simulink model "scattering_pos_pos_old"  (R2022b)
settings: Solver=VariableStepAuto  StartTime=0.0  StopTime=10.0  RelTol=1e-3
values from neighbouring files (symbols this model uses):
  A = 2    [scattering_params.m]    (also in scattering_params_force_pos.m = 3; scattering_params_pos_pos.m = 3)
  b = 1    [scattering_params.m]    (also in scattering_params_force_pos.m = 40; scattering_params_pos_pos.m = 100)
  Be = 100    [scattering_params.m]    (also in scattering_params_force_pos.m; scattering_params_pos_pos.m)
  Bh = 1.5    [scattering_params.m]    (also in scattering_params_force_pos.m = 1; scattering_params_pos_pos.m = 1)
  Dh = 0.1    [scattering_params.m]    (also in scattering_params_force_pos.m = 16; scattering_params_pos_pos.m = 16)
  discrete_delay = 100    [scattering_params_force_pos.m]    (also in scattering_params_pos_pos.m)
  Fc = 1    [scattering_params.m]    (also in scattering_params_force_pos.m = 0.25; scattering_params_pos_pos.m = 0.25)
  Flp = 5    [scattering_params.m]    (also in scattering_params_force_pos.m = 0.5; scattering_params_pos_pos.m = 0.5)
  Jh = 1    [scattering_params.m]    (also in scattering_params_force_pos.m; scattering_params_pos_pos.m)
  Ke = 200    [scattering_params.m]    (also in scattering_params_force_pos.m; scattering_params_pos_pos.m)
  Mm = 0.5    [scattering_params.m]    (also in scattering_params_force_pos.m; scattering_params_pos_pos.m)
  Ms = 2    [scattering_params.m]    (also in scattering_params_force_pos.m; scattering_params_pos_pos.m)
  Ph = 10    [scattering_params.m]    (also in scattering_params_force_pos.m; scattering_params_pos_pos.m)
  scattering_filter_freq = 10    [scattering_params.m]    (also in scattering_params_force_pos.m; scattering_params_pos_pos.m)
  Ts = 0.001    [scattering_params_force_pos.m]    (also in scattering_params_pos_pos.m)
  xe = 5    [scattering_params.m]    (also in scattering_params_force_pos.m = 2; scattering_params_pos_pos.m = 2)
settings Model: Creator=Manu  LastModifiedBy=Manu

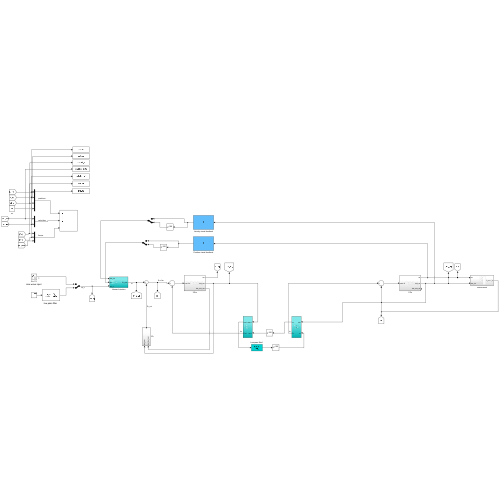
[thumbnail: Simulink's stored preview of the top-level diagram]
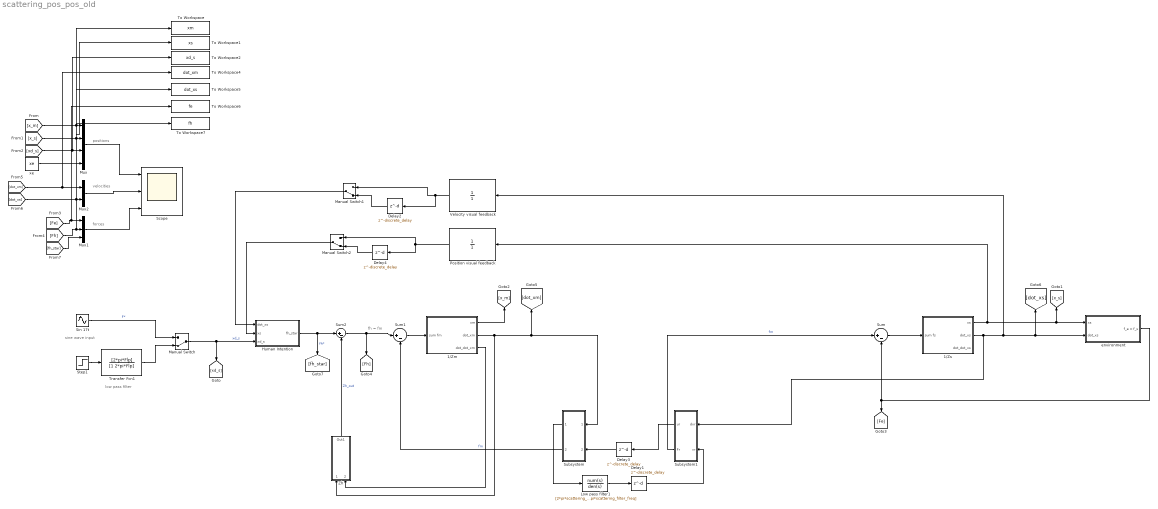
== system scattering_pos_pos_old ==
  note: fh = fm
  note: sine wave input
  note: low pass filter
  note: positions
  note: forces
  note: velocities
  1/Zm : Subsystem
  1/Zs : Subsystem
  Delay{1..4} (4 alike) : Delay  DelayLength=discrete_delay  SampleTime=Ts
  Human Intention : Subsystem
  Low pass filter1 : TransferFcn  Numerator=[2*pi*scattering_filter_freq]  Denominator=[1 2*pi*scattering_filter_freq]
  Manual Switch : ManualSwitch  CurrentSetting=0
  Manual Switch1 : ManualSwitch  CurrentSetting=0
  Manual Switch2 : ManualSwitch  CurrentSetting=0
  Mux : Mux
  Mux1 : Mux  Inputs=3
  Mux2 : Mux  Inputs=2
  Position visual feedback : TransferFcn  Denominator=[1]
  Scope : Scope  NumInputPorts=3
  Sin 17t : Sin  Amplitude=A  Frequency=2*pi*Fc  SampleTime=0
  Step1 : Step  Time=0.5  After=A  SampleTime=0
  Subsystem : Subsystem
      settings: PortSchema="{\"entries\":[{\"content\":{\"sides\":[{\"content\":{\"connectorIds\":[\"Out1\",\"Out2\"]},\"type\":\"ConnectorPlacement.EquallySpacedRectSide\",\"uuid\":\"82be490b-f4e1-4469-8bd6-488a0e070f91\"},{\"content\":{\"connectorIds\":[\"In1\",\"In2\"],\"side\":\"RIGHT\"},\"type\":\"ConnectorPlacement.EquallySpacedRectSide\",\"uuid\":\"c4a13bf6-21c5-475e-be70-cb3636e820b8\"},{\"content\":{\"connectorIds\":[],\"side\":\"TOP\"},\"type\":\"ConnectorPlacement.EquallySpacedRectSide\",\"uuid\":\"239945ea-98d9-43ca-9337-d0acd489fa2c\"},{\"content\":{\"connectorIds\":[],\"side\":\"HIDDEN\"},\"type\":\"ConnectorPlacement.EquallySpacedRectSide\",\"uuid\":\"ab55d6c9-2d6b-496a-b62d-f74546630c92\"}]},\"type\":\"ConnectorPlacement.EquallySpacedConnector\",\"uuid\":\"f2ee4140-76ed-4153-9f7f-3580e67d072a\"}],\"packageUris\":[\"http://schema.mathworks.com/mf0/Connector/R2020b\"],\"version\":\"1.0\"}"
  Subsystem1 : Subsystem
      settings: PortSchema="{\"entries\":[{\"content\":{\"sides\":[{\"content\":{\"connectorIds\":[\"Out1\",\"Out2\"]},\"type\":\"ConnectorPlacement.EquallySpacedRectSide\",\"uuid\":\"82be490b-f4e1-4469-8bd6-488a0e070f91\"},{\"content\":{\"connectorIds\":[\"In1\",\"In2\"],\"side\":\"RIGHT\"},\"type\":\"ConnectorPlacement.EquallySpacedRectSide\",\"uuid\":\"c4a13bf6-21c5-475e-be70-cb3636e820b8\"},{\"content\":{\"connectorIds\":[],\"side\":\"TOP\"},\"type\":\"ConnectorPlacement.EquallySpacedRectSide\",\"uuid\":\"239945ea-98d9-43ca-9337-d0acd489fa2c\"},{\"content\":{\"connectorIds\":[],\"side\":\"HIDDEN\"},\"type\":\"ConnectorPlacement.EquallySpacedRectSide\",\"uuid\":\"ab55d6c9-2d6b-496a-b62d-f74546630c92\"}]},\"type\":\"ConnectorPlacement.EquallySpacedConnector\",\"uuid\":\"f2ee4140-76ed-4153-9f7f-3580e67d072a\"}],\"packageUris\":[\"http://schema.mathworks.com/mf0/Connector/R2020b\"],\"version\":\"1.0\"}"
  Sum : Sum  Inputs=|+-
  Sum1 : Sum  Inputs=|+-
  Sum2 : Sum  Inputs=|+-
  To Workspace : ToWorkspace  VariableName=xm  SaveFormat=Timeseries  SampleTime=-1
  To Workspace1 : ToWorkspace  VariableName=xs  SaveFormat=Timeseries  SampleTime=-1
  To Workspace2 : ToWorkspace  VariableName=xd_s  SaveFormat=Timeseries  SampleTime=-1
  To Workspace4 : ToWorkspace  VariableName=dot_xm  SaveFormat=Timeseries  SampleTime=-1
  To Workspace5 : ToWorkspace  VariableName=dot_xs  SaveFormat=Timeseries  SampleTime=-1
  To Workspace6 : ToWorkspace  VariableName=fe  SaveFormat=Timeseries  SampleTime=-1
  To Workspace7 : ToWorkspace  VariableName=fh  SaveFormat=Timeseries  SampleTime=-1
  Transfer Fcn1 : TransferFcn  Numerator=[2*pi*Flp]  Denominator=[1 2*pi*Flp]
  Velocity visual feedback : TransferFcn  Denominator=[1]
  Zh : Subsystem
  environment : Subsystem
  xe : Constant  Value=xe
  wires:
  1/Zm/1(xm) -> [x_m]
  Manual Switch/1 -> [xd_s], Human Intention/3(xd_s)  "xd_s"
  Zh/1(Out1) -> Sum2/2  "Zh_out"
  Sin 17t/1 -> Manual Switch/1  "F*"
  1/Zm/3(dot_dot_xm) -> Zh/2(dot_dot_xm)
  Human Intention/1(fh_star) -> Sum2/1, [fh_star]  "fh*"
  Transfer Fcn1/1 -> Manual Switch/2
  Step1/1 -> Transfer Fcn1/1
  Sum2/1 -> [Fh], Sum1/1
  Sum1/1 -> 1/Zm/1(sum fm)
  Sum/1 -> 1/Zs/1(sum fs)
  1/Zs/2(dot_xs) -> Subsystem1/1(dxr), Velocity visual feedback/1, [dot_xs], environment/2(dot_xs)
  1/Zs/1(xs) -> [x_s], environment/1(xs), Position visual feedback/1
  environment/1(f_e = f_s) -> [Fe], Sum/2
  Velocity visual feedback/1 -> Delay2/1, Manual Switch1/1
  Manual Switch1/1 -> Human Intention/1(dot_xs)
  Delay4/1 -> Manual Switch2/2
  Position visual feedback/1 -> Delay4/1, Manual Switch2/1
  Manual Switch2/1 -> Human Intention/2(xs)
  1/Zm/2(dot_xm) -> Subsystem/1(dxm1), [dot_xm], Zh/1(dot_xm)
  Subsystem/2(Fm1) -> Sum1/2  "fm"
  Subsystem1/2(Fr) -> Sum/1  "fm"
  Subsystem/1(um1) -> Low pass filter1/1
  Subsystem1/1(ur) -> Delay3/1
  Low pass filter1/1 -> Delay1/1
  Delay2/1 -> Manual Switch1/2
  Delay3/1 -> Subsystem/2(vm1)
  Delay1/1 -> Subsystem1/2(vr)
  [fh_star] -> Mux1/3
  Mux2/1 -> Scope/2
  [Fh] -> To Workspace7/1, Mux1/2
  [dot_xs] -> To Workspace5/1, Mux2/2
  [dot_xm] -> Mux2/1, To Workspace4/1
  [x_s] -> To Workspace1/1, Mux/2
  [x_m] -> To Workspace/1, Mux/1
  Mux1/1 -> Scope/3
  Mux/1 -> Scope/1
  xe/1 -> Mux/4
  [Fe] -> Mux1/1, To Workspace6/1
  [xd_s] -> To Workspace2/1, Mux/3

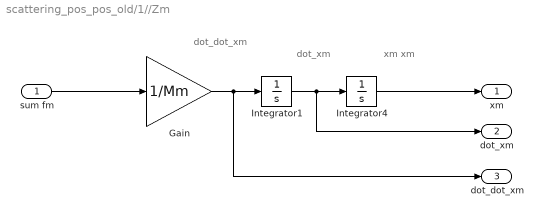
== system scattering_pos_pos_old/1//Zm ==
  note: dot_dot_xm
  note: dot_xm
  note: xm
      | xm
  sum fm : Inport
  Gain : Gain  Gain=1/Mm
  Integrator1 : Integrator
  Integrator4 : Integrator
  xm : Outport
  dot_xm : Outport  Port=2
  dot_dot_xm : Outport  Port=3
  wires:
  sum fm/1 -> Gain/1
  Gain/1 -> dot_dot_xm/1, Integrator1/1
  Integrator4/1 -> xm/1
  Integrator1/1 -> dot_xm/1, Integrator4/1

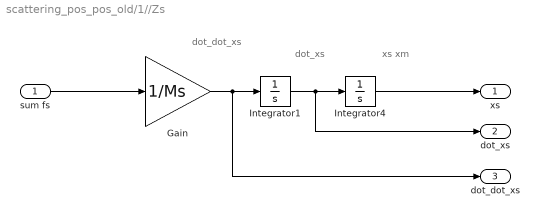
== system scattering_pos_pos_old/1//Zs ==
  note: dot_dot_xs
  note: dot_xs
  note: xs
      | xm
  sum fs : Inport
  Gain : Gain  Gain=1/Ms
  Integrator1 : Integrator
  Integrator4 : Integrator
  xs : Outport
  dot_xs : Outport  Port=2
  dot_dot_xs : Outport  Port=3
  wires:
  sum fs/1 -> Gain/1
  Gain/1 -> dot_dot_xs/1, Integrator1/1
  Integrator4/1 -> xs/1
  Integrator1/1 -> dot_xs/1, Integrator4/1

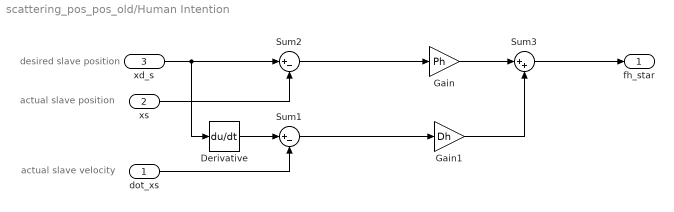
== system scattering_pos_pos_old/Human Intention ==
  note: actual slave velocity
  note: actual slave position
  note: desired slave position
  dot_xs : Inport
  xs : Inport  Port=2
  xd_s : Inport  Port=3
  Derivative : Derivative
  Gain : Gain  Gain=Ph
  Gain1 : Gain  Gain=Dh
  Sum1 : Sum  Inputs=|+-
  Sum2 : Sum  Inputs=|+-
  Sum3 : Sum  Inputs=|++
  fh_star : Outport
  wires:
  xs/1 -> Sum2/2
  dot_xs/1 -> Sum1/2
  Sum2/1 -> Gain/1
  Sum1/1 -> Gain1/1
  Gain1/1 -> Sum3/2
  Gain/1 -> Sum3/1
  Sum3/1 -> fh_star/1
  xd_s/1 -> Derivative/1, Sum2/1
  Derivative/1 -> Sum1/1

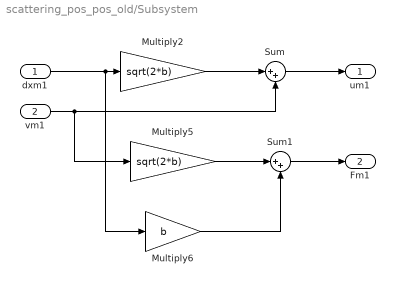
== system scattering_pos_pos_old/Subsystem ==
  dxm1 : Inport
  vm1 : Inport  Port=2
  Multiply2 : Gain  Gain=sqrt(2*b)
  Multiply5 : Gain  Gain=sqrt(2*b)
  Multiply6 : Gain  Gain=b
  Sum : Sum  Inputs=|++
  Sum1 : Sum  Inputs=|++
  um1 : Outport
  Fm1 : Outport  Port=2
  wires:
  dxm1/1 -> Multiply6/1, Multiply2/1
  vm1/1 -> Multiply5/1, Sum/2
  Multiply2/1 -> Sum/1
  Sum/1 -> um1/1
  Multiply5/1 -> Sum1/1
  Sum1/1 -> Fm1/1
  Multiply6/1 -> Sum1/2

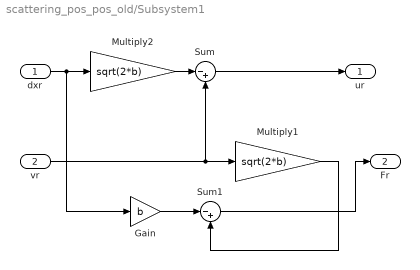
== system scattering_pos_pos_old/Subsystem1 ==
  dxr : Inport
  vr : Inport  Port=2
  Gain : Gain  Gain=b
  Multiply1 : Gain  Gain=sqrt(2*b)
  Multiply2 : Gain  Gain=sqrt(2*b)
  Sum : Sum  Inputs=|-+
  Sum1 : Sum  Inputs=|-+
  ur : Outport
  Fr : Outport  Port=2
  wires:
  dxr/1 -> Gain/1, Multiply2/1
  Multiply2/1 -> Sum/1
  vr/1 -> Multiply1/1, Sum/2
  Sum/1 -> ur/1
  Gain/1 -> Sum1/1
  Multiply1/1 -> Sum1/2
  Sum1/1 -> Fr/1

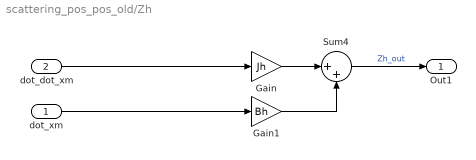
== system scattering_pos_pos_old/Zh ==
  dot_xm : Inport
  dot_dot_xm : Inport  Port=2
  Gain : Gain  Gain=Jh
  Gain1 : Gain  Gain=Bh
  Sum4 : Sum  Inputs=|++
  Out1 : Outport
  wires:
  dot_dot_xm/1 -> Gain/1
  Gain1/1 -> Sum4/2
  Gain/1 -> Sum4/1
  Sum4/1 -> Out1/1  "Zh_out"
  dot_xm/1 -> Gain1/1

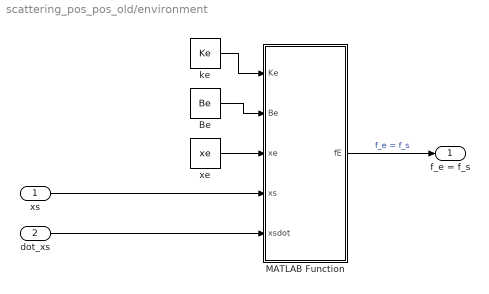
== system scattering_pos_pos_old/environment ==
  xs : Inport
  dot_xs : Inport  Port=2
  Be : Constant  Value=Be
  MATLAB Function : MATLAB Function  TreatAsAtomicUnit=on
  ke : Constant  Value=Ke
  xe : Constant  Value=xe
  f_e = f_s : Outport
  wires:
  MATLAB Function/1(fE) -> f_e = f_s/1  "f_e = f_s"
  xs/1 -> MATLAB Function/4(xs)
  xe/1 -> MATLAB Function/3(xe)
  dot_xs/1 -> MATLAB Function/5(xsdot)
  ke/1 -> MATLAB Function/1(Ke)
  Be/1 -> MATLAB Function/2(Be)

== matlab function scattering_pos_pos_old/environment/MATLAB Function ==
  data: Ke input; fE output; Be input; xe input; xs input; xsdot input
function fE = environment(Ke, Be, xe, xs, xsdot)
    if xs > xe
        fE = Ke * (xs - xe) + Be * xsdot; % Plot both contributions Ke and Be
    else
        fE = 0;
    end
end
